simulink library "inp"  (R2021b)
settings: Solver=VariableStepAuto  StartTime=0.0  StopTime=10.0  RelTol=1e-3
undefined symbols (not defined in the file): C_TASK_5MS_S, FALSE, KINP_AcoreReadyToSlp_flg_ovrdflg, KINP_AcoreReadyToSlp_flg_ovrdval, KINP_AllowMovThd_OTA_enum_ovrdflg, KINP_AllowMovThd_OTA_enum_ovrdval, KINP_APSAngleTarget_Deg_ovrdflg, KINP_APSAngleTarget_Deg_ovrdval, KINP_APSDecReq_mps2_ovrdflg, KINP_APSDecReq_mps2_ovrdval, KINP_APSDecReqA_flg_ovrdflg, KINP_APSDecReqA_flg_ovrdval, KINP_APSDFLL_cm_ovrdflg, KINP_APSDFLL_cm_ovrdval, KINP_APSDFLR_cm_ovrdflg, KINP_APSDFLR_cm_ovrdval, KINP_APSDRLL_cm_ovrdflg, KINP_APSDRLL_cm_ovrdval, KINP_APSDRLR_cm_ovrdflg, KINP_APSDRLR_cm_ovrdval, KINP_APSExitCondition_enum_ovrdflg, KINP_APSExitCondition_enum_ovrdval, KINP_APSHWVer_enum_ovrdflg, KINP_APSHWVer_enum_ovrdval, KINP_APSProgressPCT_pct_ovrdflg, KINP_APSProgressPCT_pct_ovrdval, KINP_APSPwrReq_enum_ovrdflg, KINP_APSPwrReq_enum_ovrdval, KINP_APSReq_enum_ovrdflg, KINP_APSReq_enum_ovrdval, KINP_APSRQDisplay_enum_ovrdflg, KINP_APSRQDisplay_enum_ovrdval, KINP_APSRqEPASCtrl_flg_ovrdflg, KINP_APSRqEPASCtrl_flg_ovrdval, KINP_APSShiftPosnReq_enum_ovrdval, KINP_APSShiftPosnReq_enum_ovrflg, KINP_APSSpeedCMD_kph_ovrdval, KINP_APSSpeedCMD_kph_ovrflg, KINP_APSStaSystem_enum_ovrdflg, KINP_APSStaSystem_enum_ovrdval, KINP_APSSWVer_enum_ovrdflg, KINP_APSSWVer_enum_ovrdval, KINP_APSVMCReqA_flg_ovrdval, KINP_APSVMCReqA_flg_ovrflg, KINP_APSVRqEPASCtrl_flg_ovrdflg, KINP_APSVRqEPASCtrl_flg_ovrdval, KINP_AuxBattVolmV_mV_ovrdflg, KINP_AuxBattVolmV_mV_ovrdval, KINP_BTConnectSta_enum_ovrdflg, KINP_BTConnectSta_enum_ovrdval, KINP_CAASSta_enum_ovrdflg, KINP_CAASSta_enum_ovrdval, KINP_CAASVMCReqA_flg_ovrdval, KINP_CAASVMCReqA_flg_ovrflg, KINP_CAN1BusOff_flg_ovrdflg, KINP_CAN1BusOff_flg_ovrdval, KINP_CAN2BusOff_flg_ovrdflg, KINP_CAN2BusOff_flg_ovrdval, KINP_CAN3BusOff_flg_ovrdflg, KINP_CAN3BusOff_flg_ovrdval ... (+158)
libraries: FVT_lib x184, hcu_lib x1
(part 4 of 8)

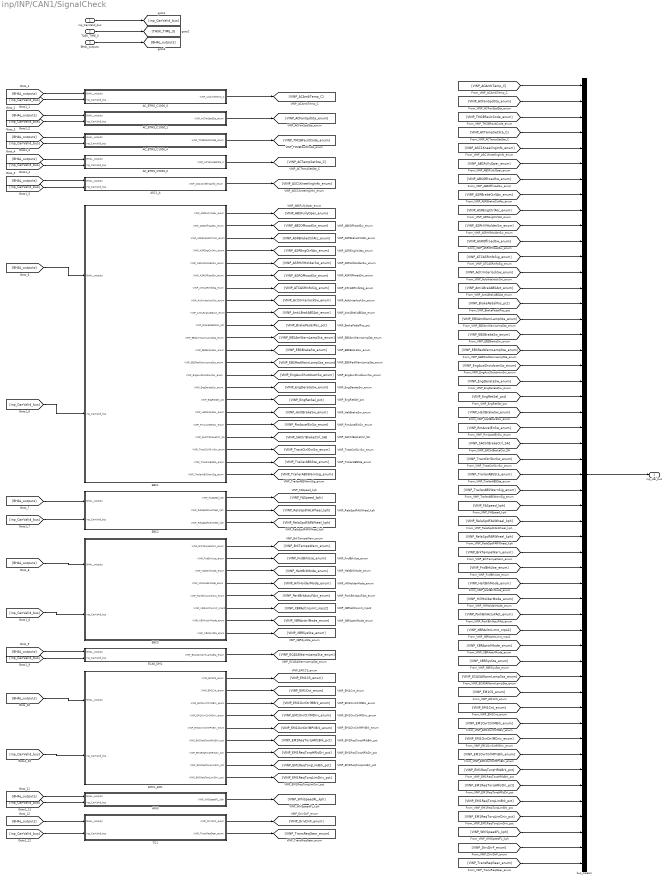
== system inp/INP/CAN1/SignalCheck ==
  inp_CanValid_bus : Inport
  TASK_TIME_S : Inport  Port=2
  BHAL_outputs : Inport  Port=3
  AC_BTMS_C1000_0 : Subsystem
  AC_BTMS_C1000_1 : Subsystem
  AC_BTMS_C1000_4 : Subsystem
  AC_BTMS_C5000_0 : Subsystem
  ASC1_A : Subsystem
  EBC1 : Subsystem
  EBC2 : Subsystem
  EBC5 : Subsystem
  ECAS_DM1 : Subsystem
  EMC1_EM1 : Subsystem
  HRW : Subsystem
  TC1 : Subsystem
  bus_creator : BusCreator  Inputs=51
  inp_Hal_bus : Outport
  wires:
  inp_CanValid_bus/1 -> [inp_CanValid_bus]
  TASK_TIME_S/1 -> [TASK_TIME_S]
  BHAL_outputs/1 -> [BHAL_outputs]
  [BHAL_outputs] -> AC_BTMS_C1000_0/1(BHAL_outputs)
  [inp_CanValid_bus] -> AC_BTMS_C1000_0/2(inp_CanValid_bus)
  AC_BTMS_C1000_0/1(VINP_ACAmbTemp_C) -> [VINP_ACAmbTemp_C]
  [BHAL_outputs] -> AC_BTMS_C1000_1/1(BHAL_outputs)
  [inp_CanValid_bus] -> AC_BTMS_C1000_1/2(inp_CanValid_bus)
  AC_BTMS_C1000_1/1(VINP_ACFanSpdSta_enum) -> [VINP_ACFanSpdSta_enum]
  [BHAL_outputs] -> AC_BTMS_C1000_4/1(BHAL_outputs)
  [inp_CanValid_bus] -> AC_BTMS_C1000_4/2(inp_CanValid_bus)
  AC_BTMS_C1000_4/1(VINP_TM2BFaultCode_enum) -> [VINP_TM2BFaultCode_enum]
  [BHAL_outputs] -> AC_BTMS_C5000_0/1(BHAL_outputs)
  [inp_CanValid_bus] -> AC_BTMS_C5000_0/2(inp_CanValid_bus)
  AC_BTMS_C5000_0/1(VINP_ACTempSetSta_C) -> [VINP_ACTempSetSta_C]
  [BHAL_outputs] -> ASC1_A/1(BHAL_outputs)
  [inp_CanValid_bus] -> ASC1_A/2(inp_CanValid_bus)
  ASC1_A/1(VINP_ASC1KneelingInfo_enum) -> [VINP_ASC1KneelingInfo_enum]
  [BHAL_outputs] -> EBC1/1(BHAL_outputs)
  [inp_CanValid_bus] -> EBC1/2(inp_CanValid_bus)
  EBC1/1(VINP_ABSFullyOper_enum) -> [VINP_ABSFullyOper_enum]
  EBC1/2(VINP_ABSOffroadSw_enum) -> [VINP_ABSOffroadSw_enum]
  EBC1/3(VINP_ASRBrakeCtrlAtc_enum) -> [VINP_ASRBrakeCtrlAtc_enum]
  EBC1/4(VINP_ASREngCtrlAtc_enum) -> [VINP_ASREngCtrlAtc_enum]
  EBC1/5(VINP_ASRHillHolderSw_enum) -> [VINP_ASRHillHolderSw_enum]
  EBC1/6(VINP_ASROffroadSw_enum) -> [VINP_ASROffroadSw_enum]
  EBC1/7(VINP_ATCASRInfoSig_enum) -> [VINP_ATCASRInfoSig_enum]
  EBC1/8(VINP_AcltrInterlockSw_enum) -> [VINP_AcltrInterlockSw_enum]
  EBC1/9(VINP_AntiLBrakABSAct_enum) -> [VINP_AntiLBrakABSAct_enum]
  EBC1/10(VINP_BrakePedalPos_pct) -> [VINP_BrakePedalPos_pct]
  EBC1/11(VINP_EBSAmWarnLampSta_enum) -> [VINP_EBSAmWarnLampSta_enum]
  EBC1/12(VINP_EBSBrakeSw_enum) -> [VINP_EBSBrakeSw_enum]
  EBC1/13(VINP_EBSRedWarnLampSta_enum) -> [VINP_EBSRedWarnLampSta_enum]
  EBC1/14(VINP_EngAuxShutdownSw_enum) -> [VINP_EngAuxShutdownSw_enum]
  EBC1/15(VINP_EngDerateSw_enum) -> [VINP_EngDerateSw_enum]
  EBC1/16(VINP_EngRetSel_pct) -> [VINP_EngRetSel_pct]
  EBC1/17(VINP_HaltBrakeSw_enum) -> [VINP_HaltBrakeSw_enum]
  EBC1/18(VINP_RmAccelEnSw_enum) -> [VINP_RmAccelEnSw_enum]
  EBC1/19(VINP_SACtrlBrakeCtrl_SA) -> [VINP_SACtrlBrakeCtrl_SA]
  EBC1/20(VINP_TractCtrlOvrSw_enum) -> [VINP_TractCtrlOvrSw_enum]
  EBC1/21(VINP_TrailerABSSta_enum) -> [VINP_TrailerABSSta_enum]
  EBC1/22(VINP_TrailerABSWarnSig_enum) -> [VINP_TrailerABSWarnSig_enum]
  [BHAL_outputs] -> EBC2/1(BHAL_outputs)
  [inp_CanValid_bus] -> EBC2/2(inp_CanValid_bus)
  EBC2/1(VINP_FASpeed_kph) -> [VINP_FASpeed_kph]
  EBC2/2(VINP_RelaSpdFALWheel_kph) -> [VINP_RelaSpdFALWheel_kph]
  EBC2/3(VINP_RelaSpdFARWheel_kph) -> [VINP_RelaSpdFARWheel_kph]
  [BHAL_outputs] -> EBC5/1(BHAL_outputs)
  [inp_CanValid_bus] -> EBC5/2(inp_CanValid_bus)
  EBC5/1(VINP_BrkTempeWarn_enum) -> [VINP_BrkTempeWarn_enum]
  EBC5/2(VINP_FndBrkUse_enum) -> [VINP_FndBrkUse_enum]
  EBC5/3(VINP_HaltBrkMode_enum) -> [VINP_HaltBrkMode_enum]
  EBC5/4(VINP_HillHolderMode_enum) -> [VINP_HillHolderMode_enum]
  EBC5/5(VINP_ParkBrkActuFAct_enum) -> [VINP_ParkBrkActuFAct_enum]
  EBC5/6(VINP_XBRAcltnLimit_mps2) -> [VINP_XBRAcltnLimit_mps2]
  EBC5/7(VINP_XBRActtrlMode_enum) -> [VINP_XBRActtrlMode_enum]
  EBC5/8(VINP_XBRSysSta_enum) -> [VINP_XBRSysSta_enum]
  [BHAL_outputs] -> ECAS_DM1/1(BHAL_outputs)
  [inp_CanValid_bus] -> ECAS_DM1/2(inp_CanValid_bus)
  ECAS_DM1/1(VINP_ECASAWarmLampSta_enum) -> [VINP_ECASAWarmLampSta_enum]
  [BHAL_outputs] -> EMC1_EM1/1(BHAL_outputs)
  [inp_CanValid_bus] -> EMC1_EM1/2(inp_CanValid_bus)
  EMC1_EM1/1(VINP_EM1CS_enum) -> [VINP_EM1CS_enum]
  EMC1_EM1/2(VINP_EM1Cnt_enum) -> [VINP_EM1Cnt_enum]
  EMC1_EM1/3(VINP_EM1OvrCtrlMBrk_enum) -> [VINP_EM1OvrCtrlMBrk_enum]
  EMC1_EM1/4(VINP_EM1OvrCtrlMDriv_enum) -> [VINP_EM1OvrCtrlMDriv_enum]
  EMC1_EM1/5(VINP_EM1OvrCtrlMPriBrk_enum) -> [VINP_EM1OvrCtrlMPriBrk_enum]
  EMC1_EM1/6(VINP_EM1ReqTorqHRlsBrk_pct) -> [VINP_EM1ReqTorqHRlsBrk_pct]
  EMC1_EM1/7(VINP_EM1ReqTorqHRlsDri_pct) -> [VINP_EM1ReqTorqHRlsDri_pct]
  EMC1_EM1/8(VINP_EM1ReqTorqLimBrk_pct) -> [VINP_EM1ReqTorqLimBrk_pct]
  EMC1_EM1/9(VINP_EM1ReqTorqLimDriv_pct) -> [VINP_EM1ReqTorqLimDriv_pct]
  [BHAL_outputs] -> HRW/1(BHAL_outputs)
  [inp_CanValid_bus] -> HRW/2(inp_CanValid_bus)
  HRW/1(VINP_WhlSpeedFL_kph) -> [VINP_WhlSpeedFL_kph]
  [BHAL_outputs] -> TC1/1(BHAL_outputs)
  [inp_CanValid_bus] -> TC1/2(inp_CanValid_bus)
  TC1/1(VINP_DrivDirF_enum) -> [VINP_DrivDirF_enum]
  TC1/2(VINP_TransReqGear_enum) -> [VINP_TransReqGear_enum]
  bus_creator/1 -> inp_Hal_bus/1
  [VINP_ACAmbTemp_C] -> bus_creator/1
  [VINP_ACFanSpdSta_enum] -> bus_creator/2
  [VINP_TM2BFaultCode_enum] -> bus_creator/3
  [VINP_ACTempSetSta_C] -> bus_creator/4
  [VINP_ASC1KneelingInfo_enum] -> bus_creator/5
  [VINP_ABSFullyOper_enum] -> bus_creator/6
  [VINP_ABSOffroadSw_enum] -> bus_creator/7
  [VINP_ASRBrakeCtrlAtc_enum] -> bus_creator/8
  [VINP_ASREngCtrlAtc_enum] -> bus_creator/9
  [VINP_ASRHillHolderSw_enum] -> bus_creator/10
  [VINP_ASROffroadSw_enum] -> bus_creator/11
  [VINP_ATCASRInfoSig_enum] -> bus_creator/12
  [VINP_AcltrInterlockSw_enum] -> bus_creator/13
  [VINP_AntiLBrakABSAct_enum] -> bus_creator/14
  [VINP_BrakePedalPos_pct] -> bus_creator/15
  [VINP_EBSAmWarnLampSta_enum] -> bus_creator/16
  [VINP_EBSBrakeSw_enum] -> bus_creator/17
  [VINP_EBSRedWarnLampSta_enum] -> bus_creator/18
  [VINP_EngAuxShutdownSw_enum] -> bus_creator/19
  [VINP_EngDerateSw_enum] -> bus_creator/20
  [VINP_EngRetSel_pct] -> bus_creator/21
  [VINP_HaltBrakeSw_enum] -> bus_creator/22
  [VINP_RmAccelEnSw_enum] -> bus_creator/23
  [VINP_SACtrlBrakeCtrl_SA] -> bus_creator/24
  [VINP_TractCtrlOvrSw_enum] -> bus_creator/25
  [VINP_TrailerABSSta_enum] -> bus_creator/26
  [VINP_TrailerABSWarnSig_enum] -> bus_creator/27
  [VINP_FASpeed_kph] -> bus_creator/28
  [VINP_RelaSpdFALWheel_kph] -> bus_creator/29
  [VINP_RelaSpdFARWheel_kph] -> bus_creator/30
  [VINP_BrkTempeWarn_enum] -> bus_creator/31
  [VINP_FndBrkUse_enum] -> bus_creator/32
  [VINP_HaltBrkMode_enum] -> bus_creator/33
  [VINP_HillHolderMode_enum] -> bus_creator/34
  [VINP_ParkBrkActuFAct_enum] -> bus_creator/35
  [VINP_XBRAcltnLimit_mps2] -> bus_creator/36
  [VINP_XBRActtrlMode_enum] -> bus_creator/37
  [VINP_XBRSysSta_enum] -> bus_creator/38
  [VINP_ECASAWarmLampSta_enum] -> bus_creator/39
  [VINP_EM1CS_enum] -> bus_creator/40
  [VINP_EM1Cnt_enum] -> bus_creator/41
  [VINP_EM1OvrCtrlMBrk_enum] -> bus_creator/42
  [VINP_EM1OvrCtrlMDriv_enum] -> bus_creator/43
  [VINP_EM1OvrCtrlMPriBrk_enum] -> bus_creator/44
  [VINP_EM1ReqTorqHRlsBrk_pct] -> bus_creator/45
  [VINP_EM1ReqTorqHRlsDri_pct] -> bus_creator/46
  [VINP_EM1ReqTorqLimBrk_pct] -> bus_creator/47
  [VINP_EM1ReqTorqLimDriv_pct] -> bus_creator/48
  [VINP_WhlSpeedFL_kph] -> bus_creator/49
  [VINP_DrivDirF_enum] -> bus_creator/50
  [VINP_TransReqGear_enum] -> bus_creator/51

== system inp/INP/CAN2/CommunicationCheck ==
  BHAL_outputs : Inport
  CANMsgInvalidIVIC1000 : FVT_lib/inp/CAN_Msg_Validity_Process_template  SystemSampleTime=-1  VariantActivationTime=update diagram  Latency=0  AutoFrameSizeCalculation=off
      link override ovrdflg: Value=KINP_CANMsgInvalidIVIC1000_flg_ovrdflg
      link override ovrdval: Value=KINP_CANMsgInvalidIVIC1000_flg_ovrdval
  bus_creator : BusCreator  Inputs=1
  bus_selector : BusSelector  OutputSignals=VHAL_CANMsgInvalidIVIC1000_flg
  not1 : Logic  Operator=NOT  AllPortsSameDT=off  OutDataTypeStr=boolean
  inp_CanValid_bus : Outport
  wires:
  BHAL_outputs/1 -> [BHAL_outputs]
  bus_selector/1 -> CANMsgInvalidIVIC1000/1  "<VHAL_CANMsgInvalidIVIC1000_flg>"
  CANMsgInvalidIVIC1000/1 -> not1/1
  not1/1 -> bus_creator/1  "VINP_CANMsgValidIVIC1000_flg"
  [BHAL_outputs] -> bus_selector/1
  bus_creator/1 -> inp_CanValid_bus/1

== system inp/INP/CAN2/CreateBus ==
  inp_CanValid_bus : Inport
  inp_Hal_bus : Inport  Port=2
  UnitConverter_1 : DataTypeConversion  OutDataTypeStr=boolean
  UnitConverter_2 : DataTypeConversion  OutDataTypeStr=uint8
  bus_creator : BusCreator  Inputs=2  OutDataTypeStr=Bus: BINP_CAN2_outputs  NonVirtualBus=on
  bus_selector : BusSelector  OutputSignals=VINP_CANMsgValidIVIC1000_flg
  bus_selector_1 : BusSelector  OutputSignals=VINP_IVIACFanSpdReqCmd_enum
  BINP_outputs : Outport
  wires:
  inp_CanValid_bus/1 -> [inp_CanValid_bus]
  inp_Hal_bus/1 -> [inp_Hal_bus]
  bus_selector/1 -> UnitConverter_1/1  "<VINP_CANMsgValidIVIC1000_flg>"
  UnitConverter_1/1 -> bus_creator/1  "VINP_CANMsgValidIVIC1000_flg"
  bus_selector_1/1 -> UnitConverter_2/1  "<VINP_IVIACFanSpdReqCmd_enum>"
  UnitConverter_2/1 -> bus_creator/2  "VINP_IVIACFanSpdReqCmd_enum"
  [inp_CanValid_bus] -> bus_selector/1
  [inp_Hal_bus] -> bus_selector_1/1
  bus_creator/1 -> BINP_outputs/1

== system inp/INP/CAN2/SignalCheck ==
  inp_CanValid_bus : Inport
  TASK_TIME_S : Inport  Port=2
  BHAL_outputs : Inport  Port=3
  IVI_C100_0 : Subsystem
  bus_creator : BusCreator  Inputs=1
  inp_Hal_bus : Outport
  wires:
  inp_CanValid_bus/1 -> [inp_CanValid_bus]
  TASK_TIME_S/1 -> [TASK_TIME_S]
  BHAL_outputs/1 -> [BHAL_outputs]
  [BHAL_outputs] -> IVI_C100_0/1(BHAL_outputs)
  [inp_CanValid_bus] -> IVI_C100_0/2(inp_CanValid_bus)
  IVI_C100_0/1(VINP_IVIACFanSpdReqCmd_enum) -> [VINP_IVIACFanSpdReqCmd_enum]
  bus_creator/1 -> inp_Hal_bus/1
  [VINP_IVIACFanSpdReqCmd_enum] -> bus_creator/1

== system inp/INP/CAN3/CommunicationCheck ==
  BHAL_outputs : Inport
  CANMsgInvalidB2TMInfo : FVT_lib/inp/CAN_Msg_Validity_Process_template  SystemSampleTime=-1  VariantActivationTime=update diagram  Latency=0  AutoFrameSizeCalculation=off
      link override ovrdflg: Value=KINP_CANMsgInvalidB2TMInfo_flg_ovrdflg
      link override ovrdval: Value=KINP_CANMsgInvalidB2TMInfo_flg_ovrdval
  CANMsgInvalidB2VBattInfo1 : FVT_lib/inp/CAN_Msg_Validity_Process_template  SystemSampleTime=-1  VariantActivationTime=update diagram  Latency=0  AutoFrameSizeCalculation=off
      link override ovrdflg: Value=KINP_CANMsgInvalidB2VBattInfo1_flg_ovrdflg
      link override ovrdval: Value=KINP_CANMsgInvalidB2VBattInfo1_flg_ovrdval
  CANMsgInvalidB2VCurrentLimit : FVT_lib/inp/CAN_Msg_Validity_Process_template  SystemSampleTime=-1  VariantActivationTime=update diagram  Latency=0  AutoFrameSizeCalculation=off
      link override ovrdflg: Value=KINP_CANMsgInvalidB2VCurrentLimit_flg_ovrdflg
      link override ovrdval: Value=KINP_CANMsgInvalidB2VCurrentLimit_flg_ovrdval
  CANMsgInvalidB2VFult132960 : FVT_lib/inp/CAN_Msg_Validity_Process_template  SystemSampleTime=-1  VariantActivationTime=update diagram  Latency=0  AutoFrameSizeCalculation=off
      link override ovrdflg: Value=KINP_CANMsgInvalidB2VFult132960_flg_ovrdflg
      link override ovrdval: Value=KINP_CANMsgInvalidB2VFult132960_flg_ovrdval
  CANMsgInvalidB2VST1 : FVT_lib/inp/CAN_Msg_Validity_Process_template  SystemSampleTime=-1  VariantActivationTime=update diagram  Latency=0  AutoFrameSizeCalculation=off
      link override ovrdflg: Value=KINP_CANMsgInvalidB2VST1_flg_ovrdflg
      link override ovrdval: Value=KINP_CANMsgInvalidB2VST1_flg_ovrdval
  CANMsgInvalidB2VST2 : FVT_lib/inp/CAN_Msg_Validity_Process_template  SystemSampleTime=-1  VariantActivationTime=update diagram  Latency=0  AutoFrameSizeCalculation=off
      link override ovrdflg: Value=KINP_CANMsgInvalidB2VST2_flg_ovrdflg
      link override ovrdval: Value=KINP_CANMsgInvalidB2VST2_flg_ovrdval
  CANMsgInvalidB2VST4 : FVT_lib/inp/CAN_Msg_Validity_Process_template  SystemSampleTime=-1  VariantActivationTime=update diagram  Latency=0  AutoFrameSizeCalculation=off
      link override ovrdflg: Value=KINP_CANMsgInvalidB2VST4_flg_ovrdflg
      link override ovrdval: Value=KINP_CANMsgInvalidB2VST4_flg_ovrdval
  CANMsgInvalidB2VST5 : FVT_lib/inp/CAN_Msg_Validity_Process_template  SystemSampleTime=-1  VariantActivationTime=update diagram  Latency=0  AutoFrameSizeCalculation=off
      link override ovrdflg: Value=KINP_CANMsgInvalidB2VST5_flg_ovrdflg
      link override ovrdval: Value=KINP_CANMsgInvalidB2VST5_flg_ovrdval
  CANMsgInvalidEWP1 : FVT_lib/inp/CAN_Msg_Validity_Process_template  SystemSampleTime=-1  VariantActivationTime=update diagram  Latency=0  AutoFrameSizeCalculation=off
      link override ovrdflg: Value=KINP_CANMsgInvalidEWP1_flg_ovrdflg
      link override ovrdval: Value=KINP_CANMsgInvalidEWP1_flg_ovrdval
  CANMsgInvalidTMMCUSta1 : FVT_lib/inp/CAN_Msg_Validity_Process_template  SystemSampleTime=-1  VariantActivationTime=update diagram  Latency=0  AutoFrameSizeCalculation=off
      link override ovrdflg: Value=KINP_CANMsgInvalidTMMCUSta1_flg_ovrdflg
      link override ovrdval: Value=KINP_CANMsgInvalidTMMCUSta1_flg_ovrdval
  CANMsgInvalidTMMCUSta2 : FVT_lib/inp/CAN_Msg_Validity_Process_template  SystemSampleTime=-1  VariantActivationTime=update diagram  Latency=0  AutoFrameSizeCalculation=off
      link override ovrdflg: Value=KINP_CANMsgInvalidTMMCUSta2_flg_ovrdflg
      link override ovrdval: Value=KINP_CANMsgInvalidTMMCUSta2_flg_ovrdval
  CANMsgInvalidTMMCUSta3 : FVT_lib/inp/CAN_Msg_Validity_Process_template  SystemSampleTime=-1  VariantActivationTime=update diagram  Latency=0  AutoFrameSizeCalculation=off
      link override ovrdflg: Value=KINP_CANMsgInvalidTMMCUSta3_flg_ovrdflg
      link override ovrdval: Value=KINP_CANMsgInvalidTMMCUSta3_flg_ovrdval
  bus_creator : BusCreator  Inputs=12
  bus_selector : BusSelector  OutputSignals=VHAL_CANMsgInvalidB2TMInfo_flg,VHAL_CANMsgInvalidB2VBattInfo1_flg,VHAL_CANMsgInvalidB2VCurrentLimit_flg,VHAL_CANMsgInvalidB2VFult132960_flg,VHAL_CANMsgInvalidB2VST1_flg,VHAL_CANMsgInvalidB2VST2_flg,VHAL_CANMsgInvalidB2VST4_flg,VHAL_CANMsgInvalidB2VST5_flg,VHAL_CANMsgInvalidEWP1_flg,VHAL_CANMsgInvalidTMMCUSta1_flg,VHAL_CANMsgInvalidTMMCUSta2_flg,VHAL_CANMsgInvalidTMMCUSta3_flg
  not{1..12} (12 alike) : Logic  Operator=NOT  AllPortsSameDT=off  OutDataTypeStr=boolean
  inp_CanValid_bus : Outport
  wires:
  BHAL_outputs/1 -> [BHAL_outputs]
  bus_selector/1 -> CANMsgInvalidB2TMInfo/1  "<VHAL_CANMsgInvalidB2TMInfo_flg>"
  CANMsgInvalidB2TMInfo/1 -> not1/1
  not1/1 -> bus_creator/1  "VINP_CANMsgValidB2TMInfo_flg"
  bus_selector/2 -> CANMsgInvalidB2VBattInfo1/1  "<VHAL_CANMsgInvalidB2VBattInfo1_flg>"
  CANMsgInvalidB2VBattInfo1/1 -> not2/1
  not2/1 -> bus_creator/2  "VINP_CANMsgValidB2VBattInfo1_flg"
  bus_selector/3 -> CANMsgInvalidB2VCurrentLimit/1  "<VHAL_CANMsgInvalidB2VCurrentLimit_flg>"
  CANMsgInvalidB2VCurrentLimit/1 -> not3/1
  not3/1 -> bus_creator/3  "VINP_CANMsgValidB2VCurrentLimit_flg"
  bus_selector/4 -> CANMsgInvalidB2VFult132960/1  "<VHAL_CANMsgInvalidB2VFult132960_flg>"
  CANMsgInvalidB2VFult132960/1 -> not4/1
  not4/1 -> bus_creator/4  "VINP_CANMsgValidB2VFult132960_flg"
  bus_selector/5 -> CANMsgInvalidB2VST1/1  "<VHAL_CANMsgInvalidB2VST1_flg>"
  CANMsgInvalidB2VST1/1 -> not5/1
  not5/1 -> bus_creator/5  "VINP_CANMsgValidB2VST1_flg"
  bus_selector/6 -> CANMsgInvalidB2VST2/1  "<VHAL_CANMsgInvalidB2VST2_flg>"
  CANMsgInvalidB2VST2/1 -> not6/1
  not6/1 -> bus_creator/6  "VINP_CANMsgValidB2VST2_flg"
  bus_selector/7 -> CANMsgInvalidB2VST4/1  "<VHAL_CANMsgInvalidB2VST4_flg>"
  CANMsgInvalidB2VST4/1 -> not7/1
  not7/1 -> bus_creator/7  "VINP_CANMsgValidB2VST4_flg"
  bus_selector/8 -> CANMsgInvalidB2VST5/1  "<VHAL_CANMsgInvalidB2VST5_flg>"
  CANMsgInvalidB2VST5/1 -> not8/1
  not8/1 -> bus_creator/8  "VINP_CANMsgValidB2VST5_flg"
  bus_selector/9 -> CANMsgInvalidEWP1/1  "<VHAL_CANMsgInvalidEWP1_flg>"
  CANMsgInvalidEWP1/1 -> not9/1
  not9/1 -> bus_creator/9  "VINP_CANMsgValidEWP1_flg"
  bus_selector/10 -> CANMsgInvalidTMMCUSta1/1  "<VHAL_CANMsgInvalidTMMCUSta1_flg>"
  CANMsgInvalidTMMCUSta1/1 -> not10/1
  not10/1 -> bus_creator/10  "VINP_CANMsgValidTMMCUSta1_flg"
  bus_selector/11 -> CANMsgInvalidTMMCUSta2/1  "<VHAL_CANMsgInvalidTMMCUSta2_flg>"
  CANMsgInvalidTMMCUSta2/1 -> not11/1
  not11/1 -> bus_creator/11  "VINP_CANMsgValidTMMCUSta2_flg"
  bus_selector/12 -> CANMsgInvalidTMMCUSta3/1  "<VHAL_CANMsgInvalidTMMCUSta3_flg>"
  CANMsgInvalidTMMCUSta3/1 -> not12/1
  not12/1 -> bus_creator/12  "VINP_CANMsgValidTMMCUSta3_flg"
  [BHAL_outputs] -> bus_selector/1
  bus_creator/1 -> inp_CanValid_bus/1

== system inp/INP/CAN3/CreateBus ==
  inp_CanValid_bus : Inport
  inp_Hal_bus : Inport  Port=2
  UnitConverter_{1..12,17..18,37,39} (16 alike) : DataTypeConversion  OutDataTypeStr=boolean
  UnitConverter_{13..14,19..29,32,34,36,38,42,49} (19 alike) : DataTypeConversion  OutDataTypeStr=uint8
  UnitConverter_{15..16,30..31,33,35,40..41,43..48} (14 alike) : DataTypeConversion  OutDataTypeStr=single
  bus_creator : BusCreator  Inputs=49  OutDataTypeStr=Bus: BINP_CAN3_outputs  NonVirtualBus=on
  bus_selector : BusSelector  OutputSignals=VINP_CANMsgValidB2TMInfo_flg,VINP_CANMsgValidB2VBattInfo1_flg,VINP_CANMsgValidB2VCurrentLimit_flg,VINP_CANMsgValidB2VFult132960_flg,VINP_CANMsgValidB2VST1_flg,VINP_CANMsgValidB2VST2_flg,VINP_CANMsgValidB2VST4_flg,VINP_CANMsgValidB2VST5_flg,VINP_CANMsgValidEWP1_flg,VINP_CANMsgValidTMMCUSta1_flg,VINP_CANMsgValidTMMCUSta2_flg,VINP_CANMsgValidTMMCUSta3_flg
  bus_selector_1 : BusSelector  OutputSignals=VINP_B2THVRlySta_enum,VINP_B2VBI1BattType_enum,VINP_B2VAPlsDischgCurr_A,VINP_B2VAvaPlsChgCurr_A,VINP_B2VHVILFault_flg,VINP_B2VACChgConnSta_flg,VINP_B2VACChgNegRlySta_enum,VINP_B2VACChgPosRlySta_enum,VINP_B2VBMUHVSta_enum,VINP_B2VChgMode_enum,VINP_B2VChgSta_enum,VINP_B2VDCChgConnSta_enum,VINP_B2VDCChgN1RlySta_enum,VINP_B2VDCChgP1RlySta_enum,VINP_B2VMainNegRlySta_enum,VINP_B2VFaultCode_enum,VINP_B2VFaultLv_enum,VINP_B2VPackCurr_A,VINP_B2VPackInsideVol_V,VINP_B2VRqHVPwrOff_enum,VINP_B2VSOC_pct,VINP_B2VMinTempPos_enum,VINP_B2VCellMinVol_V,VINP_EWPPEFault_enum,VINP_AtvDisChgEnFbk_flg,VINP_MCUCtrlMdSta_enum,VINP_MCUIGBTEnFbk_flg,VINP_MotorSpd_rpm,VINP_MotorTrq_Nm,VINP_MCUFailGrade_enum,VINP_MCUTemp_C,VINP_MCUTrqLimHi_Nm,VINP_MCUTrqLimLo_Nm,VINP_MotorTemp_C,VINP_MCUDCCur_A,VINP_MCUDCVol_V,VINP_MCUFailCode_enum
  BINP_outputs : Outport
  wires:
  inp_CanValid_bus/1 -> [inp_CanValid_bus]
  inp_Hal_bus/1 -> [inp_Hal_bus]
  bus_selector/1 -> UnitConverter_1/1  "<VINP_CANMsgValidB2TMInfo_flg>"
  UnitConverter_1/1 -> bus_creator/1  "VINP_CANMsgValidB2TMInfo_flg"
  bus_selector/2 -> UnitConverter_2/1  "<VINP_CANMsgValidB2VBattInfo1_flg>"
  UnitConverter_2/1 -> bus_creator/2  "VINP_CANMsgValidB2VBattInfo1_flg"
  bus_selector/3 -> UnitConverter_3/1  "<VINP_CANMsgValidB2VCurrentLimit_flg>"
  UnitConverter_3/1 -> bus_creator/3  "VINP_CANMsgValidB2VCurrentLimit_flg"
  bus_selector/4 -> UnitConverter_4/1  "<VINP_CANMsgValidB2VFult132960_flg>"
  UnitConverter_4/1 -> bus_creator/4  "VINP_CANMsgValidB2VFult132960_flg"
  bus_selector/5 -> UnitConverter_5/1  "<VINP_CANMsgValidB2VST1_flg>"
  UnitConverter_5/1 -> bus_creator/5  "VINP_CANMsgValidB2VST1_flg"
  bus_selector/6 -> UnitConverter_6/1  "<VINP_CANMsgValidB2VST2_flg>"
  UnitConverter_6/1 -> bus_creator/6  "VINP_CANMsgValidB2VST2_flg"
  bus_selector/7 -> UnitConverter_7/1  "<VINP_CANMsgValidB2VST4_flg>"
  UnitConverter_7/1 -> bus_creator/7  "VINP_CANMsgValidB2VST4_flg"
  bus_selector/8 -> UnitConverter_8/1  "<VINP_CANMsgValidB2VST5_flg>"
  UnitConverter_8/1 -> bus_creator/8  "VINP_CANMsgValidB2VST5_flg"
  bus_selector/9 -> UnitConverter_9/1  "<VINP_CANMsgValidEWP1_flg>"
  UnitConverter_9/1 -> bus_creator/9  "VINP_CANMsgValidEWP1_flg"
  bus_selector/10 -> UnitConverter_10/1  "<VINP_CANMsgValidTMMCUSta1_flg>"
  UnitConverter_10/1 -> bus_creator/10  "VINP_CANMsgValidTMMCUSta1_flg"
  bus_selector/11 -> UnitConverter_11/1  "<VINP_CANMsgValidTMMCUSta2_flg>"
  UnitConverter_11/1 -> bus_creator/11  "VINP_CANMsgValidTMMCUSta2_flg"
  bus_selector/12 -> UnitConverter_12/1  "<VINP_CANMsgValidTMMCUSta3_flg>"
  UnitConverter_12/1 -> bus_creator/12  "VINP_CANMsgValidTMMCUSta3_flg"
  bus_selector_1/1 -> UnitConverter_13/1  "<VINP_B2THVRlySta_enum>"
  UnitConverter_13/1 -> bus_creator/13  "VINP_B2THVRlySta_enum"
  bus_selector_1/2 -> UnitConverter_14/1  "<VINP_B2VBI1BattType_enum>"
  UnitConverter_14/1 -> bus_creator/14  "VINP_B2VBI1BattType_enum"
  bus_selector_1/3 -> UnitConverter_15/1  "<VINP_B2VAPlsDischgCurr_A>"
  UnitConverter_15/1 -> bus_creator/15  "VINP_B2VAPlsDischgCurr_A"
  bus_selector_1/4 -> UnitConverter_16/1  "<VINP_B2VAvaPlsChgCurr_A>"
  UnitConverter_16/1 -> bus_creator/16  "VINP_B2VAvaPlsChgCurr_A"
  bus_selector_1/5 -> UnitConverter_17/1  "<VINP_B2VHVILFault_flg>"
  UnitConverter_17/1 -> bus_creator/17  "VINP_B2VHVILFault_flg"
  bus_selector_1/6 -> UnitConverter_18/1  "<VINP_B2VACChgConnSta_flg>"
  UnitConverter_18/1 -> bus_creator/18  "VINP_B2VACChgConnSta_flg"
  bus_selector_1/7 -> UnitConverter_19/1  "<VINP_B2VACChgNegRlySta_enum>"
  UnitConverter_19/1 -> bus_creator/19  "VINP_B2VACChgNegRlySta_enum"
  bus_selector_1/8 -> UnitConverter_20/1  "<VINP_B2VACChgPosRlySta_enum>"
  UnitConverter_20/1 -> bus_creator/20  "VINP_B2VACChgPosRlySta_enum"
  bus_selector_1/9 -> UnitConverter_21/1  "<VINP_B2VBMUHVSta_enum>"
  UnitConverter_21/1 -> bus_creator/21  "VINP_B2VBMUHVSta_enum"
  bus_selector_1/10 -> UnitConverter_22/1  "<VINP_B2VChgMode_enum>"
  UnitConverter_22/1 -> bus_creator/22  "VINP_B2VChgMode_enum"
  bus_selector_1/11 -> UnitConverter_23/1  "<VINP_B2VChgSta_enum>"
  UnitConverter_23/1 -> bus_creator/23  "VINP_B2VChgSta_enum"
  bus_selector_1/12 -> UnitConverter_24/1  "<VINP_B2VDCChgConnSta_enum>"
  UnitConverter_24/1 -> bus_creator/24  "VINP_B2VDCChgConnSta_enum"
  bus_selector_1/13 -> UnitConverter_25/1  "<VINP_B2VDCChgN1RlySta_enum>"
  UnitConverter_25/1 -> bus_creator/25  "VINP_B2VDCChgN1RlySta_enum"
  bus_selector_1/14 -> UnitConverter_26/1  "<VINP_B2VDCChgP1RlySta_enum>"
  UnitConverter_26/1 -> bus_creator/26  "VINP_B2VDCChgP1RlySta_enum"
  bus_selector_1/15 -> UnitConverter_27/1  "<VINP_B2VMainNegRlySta_enum>"
  UnitConverter_27/1 -> bus_creator/27  "VINP_B2VMainNegRlySta_enum"
  bus_selector_1/16 -> UnitConverter_28/1  "<VINP_B2VFaultCode_enum>"
  UnitConverter_28/1 -> bus_creator/28  "VINP_B2VFaultCode_enum"
  bus_selector_1/17 -> UnitConverter_29/1  "<VINP_B2VFaultLv_enum>"
  UnitConverter_29/1 -> bus_creator/29  "VINP_B2VFaultLv_enum"
  bus_selector_1/18 -> UnitConverter_30/1  "<VINP_B2VPackCurr_A>"
  UnitConverter_30/1 -> bus_creator/30  "VINP_B2VPackCurr_A"
  bus_selector_1/19 -> UnitConverter_31/1  "<VINP_B2VPackInsideVol_V>"
  UnitConverter_31/1 -> bus_creator/31  "VINP_B2VPackInsideVol_V"
  bus_selector_1/20 -> UnitConverter_32/1  "<VINP_B2VRqHVPwrOff_enum>"
  UnitConverter_32/1 -> bus_creator/32  "VINP_B2VRqHVPwrOff_enum"
  bus_selector_1/21 -> UnitConverter_33/1  "<VINP_B2VSOC_pct>"
  UnitConverter_33/1 -> bus_creator/33  "VINP_B2VSOC_pct"
  bus_selector_1/22 -> UnitConverter_34/1  "<VINP_B2VMinTempPos_enum>"
  UnitConverter_34/1 -> bus_creator/34  "VINP_B2VMinTempPos_enum"
  bus_selector_1/23 -> UnitConverter_35/1  "<VINP_B2VCellMinVol_V>"
  UnitConverter_35/1 -> bus_creator/35  "VINP_B2VCellMinVol_V"
  bus_selector_1/24 -> UnitConverter_36/1  "<VINP_EWPPEFault_enum>"
  UnitConverter_36/1 -> bus_creator/36  "VINP_EWPPEFault_enum"
  bus_selector_1/25 -> UnitConverter_37/1  "<VINP_AtvDisChgEnFbk_flg>"
  UnitConverter_37/1 -> bus_creator/37  "VINP_AtvDisChgEnFbk_flg"
  bus_selector_1/26 -> UnitConverter_38/1  "<VINP_MCUCtrlMdSta_enum>"
  UnitConverter_38/1 -> bus_creator/38  "VINP_MCUCtrlMdSta_enum"
  bus_selector_1/27 -> UnitConverter_39/1  "<VINP_MCUIGBTEnFbk_flg>"
  UnitConverter_39/1 -> bus_creator/39  "VINP_MCUIGBTEnFbk_flg"
  bus_selector_1/28 -> UnitConverter_40/1  "<VINP_MotorSpd_rpm>"
  UnitConverter_40/1 -> bus_creator/40  "VINP_MotorSpd_rpm"
  bus_selector_1/29 -> UnitConverter_41/1  "<VINP_MotorTrq_Nm>"
  UnitConverter_41/1 -> bus_creator/41  "VINP_MotorTrq_Nm"
  bus_selector_1/30 -> UnitConverter_42/1  "<VINP_MCUFailGrade_enum>"
  UnitConverter_42/1 -> bus_creator/42  "VINP_MCUFailGrade_enum"
  bus_selector_1/31 -> UnitConverter_43/1  "<VINP_MCUTemp_C>"
  UnitConverter_43/1 -> bus_creator/43  "VINP_MCUTemp_C"
  bus_selector_1/32 -> UnitConverter_44/1  "<VINP_MCUTrqLimHi_Nm>"
  UnitConverter_44/1 -> bus_creator/44  "VINP_MCUTrqLimHi_Nm"
  bus_selector_1/33 -> UnitConverter_45/1  "<VINP_MCUTrqLimLo_Nm>"
  UnitConverter_45/1 -> bus_creator/45  "VINP_MCUTrqLimLo_Nm"
  bus_selector_1/34 -> UnitConverter_46/1  "<VINP_MotorTemp_C>"
  UnitConverter_46/1 -> bus_creator/46  "VINP_MotorTemp_C"
  bus_selector_1/35 -> UnitConverter_47/1  "<VINP_MCUDCCur_A>"
  UnitConverter_47/1 -> bus_creator/47  "VINP_MCUDCCur_A"
  bus_selector_1/36 -> UnitConverter_48/1  "<VINP_MCUDCVol_V>"
  UnitConverter_48/1 -> bus_creator/48  "VINP_MCUDCVol_V"
  bus_selector_1/37 -> UnitConverter_49/1  "<VINP_MCUFailCode_enum>"
  UnitConverter_49/1 -> bus_creator/49  "VINP_MCUFailCode_enum"
  [inp_CanValid_bus] -> bus_selector/1
  [inp_Hal_bus] -> bus_selector_1/1
  bus_creator/1 -> BINP_outputs/1

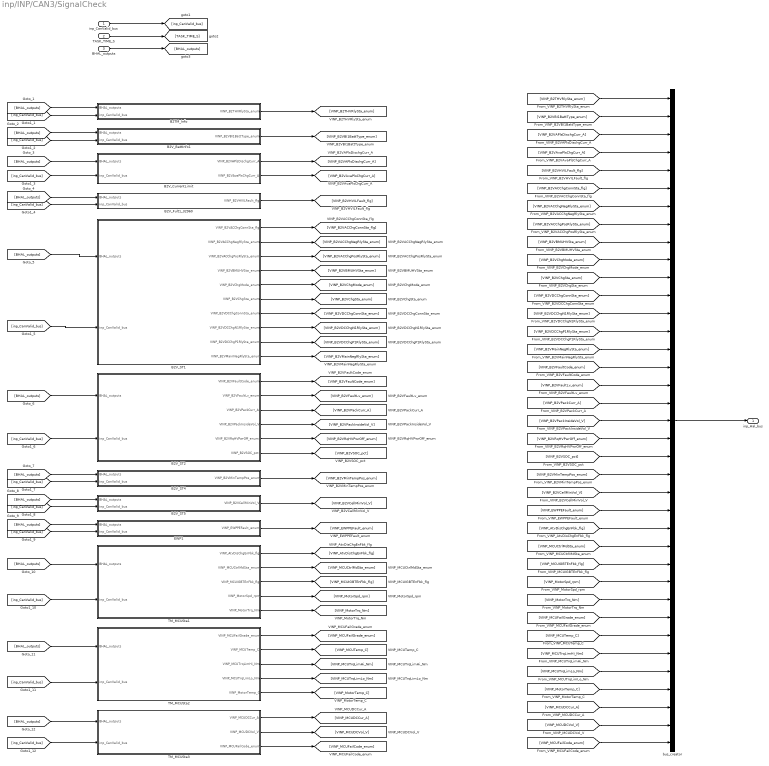
== system inp/INP/CAN3/SignalCheck ==
  inp_CanValid_bus : Inport
  TASK_TIME_S : Inport  Port=2
  BHAL_outputs : Inport  Port=3
  B2TM_Info : Subsystem
  B2V_BattInfo1 : Subsystem
  B2V_CurrentLimit : Subsystem
  B2V_Fult1_32960 : Subsystem
  B2V_ST1 : Subsystem
  B2V_ST2 : Subsystem
  B2V_ST4 : Subsystem
  B2V_ST5 : Subsystem
  EWP1 : Subsystem
  TM_MCUSta1 : Subsystem
  TM_MCUSta2 : Subsystem
  TM_MCUSta3 : Subsystem
  bus_creator : BusCreator  Inputs=37
  inp_Hal_bus : Outport
  wires:
  inp_CanValid_bus/1 -> [inp_CanValid_bus]
  TASK_TIME_S/1 -> [TASK_TIME_S]
  BHAL_outputs/1 -> [BHAL_outputs]
  [BHAL_outputs] -> B2TM_Info/1(BHAL_outputs)
  [inp_CanValid_bus] -> B2TM_Info/2(inp_CanValid_bus)
  B2TM_Info/1(VINP_B2THVRlySta_enum) -> [VINP_B2THVRlySta_enum]
  [BHAL_outputs] -> B2V_BattInfo1/1(BHAL_outputs)
  [inp_CanValid_bus] -> B2V_BattInfo1/2(inp_CanValid_bus)
  B2V_BattInfo1/1(VINP_B2VBI1BattType_enum) -> [VINP_B2VBI1BattType_enum]
  [BHAL_outputs] -> B2V_CurrentLimit/1(BHAL_outputs)
  [inp_CanValid_bus] -> B2V_CurrentLimit/2(inp_CanValid_bus)
  B2V_CurrentLimit/1(VINP_B2VAPlsDischgCurr_A) -> [VINP_B2VAPlsDischgCurr_A]
  B2V_CurrentLimit/2(VINP_B2VAvaPlsChgCurr_A) -> [VINP_B2VAvaPlsChgCurr_A]
  [BHAL_outputs] -> B2V_Fult1_32960/1(BHAL_outputs)
  [inp_CanValid_bus] -> B2V_Fult1_32960/2(inp_CanValid_bus)
  B2V_Fult1_32960/1(VINP_B2VHVILFault_flg) -> [VINP_B2VHVILFault_flg]
  [BHAL_outputs] -> B2V_ST1/1(BHAL_outputs)
  [inp_CanValid_bus] -> B2V_ST1/2(inp_CanValid_bus)
  B2V_ST1/1(VINP_B2VACChgConnSta_flg) -> [VINP_B2VACChgConnSta_flg]
  B2V_ST1/2(VINP_B2VACChgNegRlySta_enum) -> [VINP_B2VACChgNegRlySta_enum]
  B2V_ST1/3(VINP_B2VACChgPosRlySta_enum) -> [VINP_B2VACChgPosRlySta_enum]
  B2V_ST1/4(VINP_B2VBMUHVSta_enum) -> [VINP_B2VBMUHVSta_enum]
  B2V_ST1/5(VINP_B2VChgMode_enum) -> [VINP_B2VChgMode_enum]
  B2V_ST1/6(VINP_B2VChgSta_enum) -> [VINP_B2VChgSta_enum]
  B2V_ST1/7(VINP_B2VDCChgConnSta_enum) -> [VINP_B2VDCChgConnSta_enum]
  B2V_ST1/8(VINP_B2VDCChgN1RlySta_enum) -> [VINP_B2VDCChgN1RlySta_enum]
  B2V_ST1/9(VINP_B2VDCChgP1RlySta_enum) -> [VINP_B2VDCChgP1RlySta_enum]
  B2V_ST1/10(VINP_B2VMainNegRlySta_enum) -> [VINP_B2VMainNegRlySta_enum]
  [BHAL_outputs] -> B2V_ST2/1(BHAL_outputs)
  [inp_CanValid_bus] -> B2V_ST2/2(inp_CanValid_bus)
  B2V_ST2/1(VINP_B2VFaultCode_enum) -> [VINP_B2VFaultCode_enum]
  B2V_ST2/2(VINP_B2VFaultLv_enum) -> [VINP_B2VFaultLv_enum]
  B2V_ST2/3(VINP_B2VPackCurr_A) -> [VINP_B2VPackCurr_A]
  B2V_ST2/4(VINP_B2VPackInsideVol_V) -> [VINP_B2VPackInsideVol_V]
  B2V_ST2/5(VINP_B2VRqHVPwrOff_enum) -> [VINP_B2VRqHVPwrOff_enum]
  B2V_ST2/6(VINP_B2VSOC_pct) -> [VINP_B2VSOC_pct]
  [BHAL_outputs] -> B2V_ST4/1(BHAL_outputs)
  [inp_CanValid_bus] -> B2V_ST4/2(inp_CanValid_bus)
  B2V_ST4/1(VINP_B2VMinTempPos_enum) -> [VINP_B2VMinTempPos_enum]
  [BHAL_outputs] -> B2V_ST5/1(BHAL_outputs)
  [inp_CanValid_bus] -> B2V_ST5/2(inp_CanValid_bus)
  B2V_ST5/1(VINP_B2VCellMinVol_V) -> [VINP_B2VCellMinVol_V]
  [BHAL_outputs] -> EWP1/1(BHAL_outputs)
  [inp_CanValid_bus] -> EWP1/2(inp_CanValid_bus)
  EWP1/1(VINP_EWPPEFault_enum) -> [VINP_EWPPEFault_enum]
  [BHAL_outputs] -> TM_MCUSta1/1(BHAL_outputs)
  [inp_CanValid_bus] -> TM_MCUSta1/2(inp_CanValid_bus)
  TM_MCUSta1/1(VINP_AtvDisChgEnFbk_flg) -> [VINP_AtvDisChgEnFbk_flg]
  TM_MCUSta1/2(VINP_MCUCtrlMdSta_enum) -> [VINP_MCUCtrlMdSta_enum]
  TM_MCUSta1/3(VINP_MCUIGBTEnFbk_flg) -> [VINP_MCUIGBTEnFbk_flg]
  TM_MCUSta1/4(VINP_MotorSpd_rpm) -> [VINP_MotorSpd_rpm]
  TM_MCUSta1/5(VINP_MotorTrq_Nm) -> [VINP_MotorTrq_Nm]
  [BHAL_outputs] -> TM_MCUSta2/1(BHAL_outputs)
  [inp_CanValid_bus] -> TM_MCUSta2/2(inp_CanValid_bus)
  TM_MCUSta2/1(VINP_MCUFailGrade_enum) -> [VINP_MCUFailGrade_enum]
  TM_MCUSta2/2(VINP_MCUTemp_C) -> [VINP_MCUTemp_C]
  TM_MCUSta2/3(VINP_MCUTrqLimHi_Nm) -> [VINP_MCUTrqLimHi_Nm]
  TM_MCUSta2/4(VINP_MCUTrqLimLo_Nm) -> [VINP_MCUTrqLimLo_Nm]
  TM_MCUSta2/5(VINP_MotorTemp_C) -> [VINP_MotorTemp_C]
  [BHAL_outputs] -> TM_MCUSta3/1(BHAL_outputs)
  [inp_CanValid_bus] -> TM_MCUSta3/2(inp_CanValid_bus)
  TM_MCUSta3/1(VINP_MCUDCCur_A) -> [VINP_MCUDCCur_A]
  TM_MCUSta3/2(VINP_MCUDCVol_V) -> [VINP_MCUDCVol_V]
  TM_MCUSta3/3(VINP_MCUFailCode_enum) -> [VINP_MCUFailCode_enum]
  bus_creator/1 -> inp_Hal_bus/1
  [VINP_B2THVRlySta_enum] -> bus_creator/1
  [VINP_B2VBI1BattType_enum] -> bus_creator/2
  [VINP_B2VAPlsDischgCurr_A] -> bus_creator/3
  [VINP_B2VAvaPlsChgCurr_A] -> bus_creator/4
  [VINP_B2VHVILFault_flg] -> bus_creator/5
  [VINP_B2VACChgConnSta_flg] -> bus_creator/6
  [VINP_B2VACChgNegRlySta_enum] -> bus_creator/7
  [VINP_B2VACChgPosRlySta_enum] -> bus_creator/8
  [VINP_B2VBMUHVSta_enum] -> bus_creator/9
  [VINP_B2VChgMode_enum] -> bus_creator/10
  [VINP_B2VChgSta_enum] -> bus_creator/11
  [VINP_B2VDCChgConnSta_enum] -> bus_creator/12
  [VINP_B2VDCChgN1RlySta_enum] -> bus_creator/13
  [VINP_B2VDCChgP1RlySta_enum] -> bus_creator/14
  [VINP_B2VMainNegRlySta_enum] -> bus_creator/15
  [VINP_B2VFaultCode_enum] -> bus_creator/16
  [VINP_B2VFaultLv_enum] -> bus_creator/17
  [VINP_B2VPackCurr_A] -> bus_creator/18
  [VINP_B2VPackInsideVol_V] -> bus_creator/19
  [VINP_B2VRqHVPwrOff_enum] -> bus_creator/20
  [VINP_B2VSOC_pct] -> bus_creator/21
  [VINP_B2VMinTempPos_enum] -> bus_creator/22
  [VINP_B2VCellMinVol_V] -> bus_creator/23
  [VINP_EWPPEFault_enum] -> bus_creator/24
  [VINP_AtvDisChgEnFbk_flg] -> bus_creator/25
  [VINP_MCUCtrlMdSta_enum] -> bus_creator/26
  [VINP_MCUIGBTEnFbk_flg] -> bus_creator/27
  [VINP_MotorSpd_rpm] -> bus_creator/28
  [VINP_MotorTrq_Nm] -> bus_creator/29
  [VINP_MCUFailGrade_enum] -> bus_creator/30
  [VINP_MCUTemp_C] -> bus_creator/31
  [VINP_MCUTrqLimHi_Nm] -> bus_creator/32
  [VINP_MCUTrqLimLo_Nm] -> bus_creator/33
  [VINP_MotorTemp_C] -> bus_creator/34
  [VINP_MCUDCCur_A] -> bus_creator/35
  [VINP_MCUDCVol_V] -> bus_creator/36
  [VINP_MCUFailCode_enum] -> bus_creator/37

== system inp/INP/CAN4/CommunicationCheck ==
  BHAL_outputs : Inport
  CANMsgInvalidZFRC1000 : FVT_lib/inp/CAN_Msg_Validity_Process_template  SystemSampleTime=-1  VariantActivationTime=update diagram  Latency=0  AutoFrameSizeCalculation=off
      link override ovrdflg: Value=KINP_CANMsgInvalidZFRC1000_flg_ovrdflg
      link override ovrdval: Value=KINP_CANMsgInvalidZFRC1000_flg_ovrdval
  CANMsgInvalidZFRCE1000 : FVT_lib/inp/CAN_Msg_Validity_Process_template  SystemSampleTime=-1  VariantActivationTime=update diagram  Latency=0  AutoFrameSizeCalculation=off
      link override ovrdflg: Value=KINP_CANMsgInvalidZFRCE1000_flg_ovrdflg
      link override ovrdval: Value=KINP_CANMsgInvalidZFRCE1000_flg_ovrdval
  CANMsgInvalidZRRCE1000 : FVT_lib/inp/CAN_Msg_Validity_Process_template  SystemSampleTime=-1  VariantActivationTime=update diagram  Latency=0  AutoFrameSizeCalculation=off
      link override ovrdflg: Value=KINP_CANMsgInvalidZRRCE1000_flg_ovrdflg
      link override ovrdval: Value=KINP_CANMsgInvalidZRRCE1000_flg_ovrdval
  CANMsgInvalidZRRCE1001 : FVT_lib/inp/CAN_Msg_Validity_Process_template  SystemSampleTime=-1  VariantActivationTime=update diagram  Latency=0  AutoFrameSizeCalculation=off
      link override ovrdflg: Value=KINP_CANMsgInvalidZRRCE1001_flg_ovrdflg
      link override ovrdval: Value=KINP_CANMsgInvalidZRRCE1001_flg_ovrdval
  CANMsgInvalidzGWCANRr1C500 : FVT_lib/inp/CAN_Msg_Validity_Process_template  SystemSampleTime=-1  VariantActivationTime=update diagram  Latency=0  AutoFrameSizeCalculation=off
      link override ovrdflg: Value=KINP_CANMsgInvalidzGWCANRr1C500_flg_ovrdflg
      link override ovrdval: Value=KINP_CANMsgInvalidzGWCANRr1C500_flg_ovrdval
  bus_creator : BusCreator  Inputs=5
  bus_selector : BusSelector  OutputSignals=VHAL_CANMsgInvalidZFRC1000_flg,VHAL_CANMsgInvalidZFRCE1000_flg,VHAL_CANMsgInvalidZRRCE1000_flg,VHAL_CANMsgInvalidZRRCE1001_flg,VHAL_CANMsgInvalidzGWCANRr1C500_flg
  not{1..5} (5 alike) : Logic  Operator=NOT  AllPortsSameDT=off  OutDataTypeStr=boolean
  inp_CanValid_bus : Outport
  wires:
  BHAL_outputs/1 -> [BHAL_outputs]
  bus_selector/1 -> CANMsgInvalidZFRC1000/1  "<VHAL_CANMsgInvalidZFRC1000_flg>"
  CANMsgInvalidZFRC1000/1 -> not1/1
  not1/1 -> bus_creator/1  "VINP_CANMsgValidZFRC1000_flg"
  bus_selector/2 -> CANMsgInvalidZFRCE1000/1  "<VHAL_CANMsgInvalidZFRCE1000_flg>"
  CANMsgInvalidZFRCE1000/1 -> not2/1
  not2/1 -> bus_creator/2  "VINP_CANMsgValidZFRCE1000_flg"
  bus_selector/3 -> CANMsgInvalidZRRCE1000/1  "<VHAL_CANMsgInvalidZRRCE1000_flg>"
  CANMsgInvalidZRRCE1000/1 -> not3/1
  not3/1 -> bus_creator/3  "VINP_CANMsgValidZRRCE1000_flg"
  bus_selector/4 -> CANMsgInvalidZRRCE1001/1  "<VHAL_CANMsgInvalidZRRCE1001_flg>"
  CANMsgInvalidZRRCE1001/1 -> not4/1
  not4/1 -> bus_creator/4  "VINP_CANMsgValidZRRCE1001_flg"
  bus_selector/5 -> CANMsgInvalidzGWCANRr1C500/1  "<VHAL_CANMsgInvalidzGWCANRr1C500_flg>"
  CANMsgInvalidzGWCANRr1C500/1 -> not5/1
  not5/1 -> bus_creator/5  "VINP_CANMsgValidzGWCANRr1C500_flg"
  [BHAL_outputs] -> bus_selector/1
  bus_creator/1 -> inp_CanValid_bus/1

== system inp/INP/CAN4/CreateBus ==
  inp_CanValid_bus : Inport
  inp_Hal_bus : Inport  Port=2
  UnitConverter_{1..5,8..11,14,16..21,25..26,28,30..31} (21 alike) : DataTypeConversion  OutDataTypeStr=boolean
  UnitConverter_{7,12..13,15,23..24,27,29,34..35,38,41..42} (13 alike) : DataTypeConversion  OutDataTypeStr=single
  UnitConverter_{6,22,32..33,36..37,39..40,43..51} (17 alike) : DataTypeConversion  OutDataTypeStr=uint8
  bus_creator : BusCreator  Inputs=51  OutDataTypeStr=Bus: BINP_CAN4_outputs  NonVirtualBus=on
  bus_selector : BusSelector  OutputSignals=VINP_CANMsgValidZFRC1000_flg,VINP_CANMsgValidZFRCE1000_flg,VINP_CANMsgValidZRRCE1000_flg,VINP_CANMsgValidZRRCE1001_flg,VINP_CANMsgValidzGWCANRr1C500_flg
  bus_selector_1 : BusSelector  OutputSignals=VINP_ParkBrakeSW_enum,VINP_AirPressureFC2_kPa,VINP_ZFRBCMAutoLightSWSta_flg,VINP_ZFRBCMBrakeSta_flg,VINP_ZFRBCMHBeamSWSta_flg,VINP_ZFRBCMHeadLpSWSta_flg,VINP_ZFRBCMLFTurnLpCSta_A,VINP_ZFRBCMLightSensorVSta_V,VINP_ZFRBCMPLampSta_flg,VINP_ZFRBCMRFTurnLpCSta_A,VINP_ZFRBCMRFogLpSWSta_flg,VINP_ZFRBCMSeatbeltSta_flg,VINP_ZFRBCMWasherSWSta_flg,VINP_ZFRBCMWiperASSta_flg,VINP_ZFRBCMWiperHSWSta_flg,VINP_ZFRBCMWiperLSWSta_flg,VINP_ZRRBCMAllDoorSta_enum,VINP_AirPressurePC3_kPa,VINP_AirPressureRC1_kPa,VINP_FDCCHASSISVCUEACPressSta_flg,VINP_ZRRBCMCallingSWSta_flg,VINP_ZRRBCMLRTurnLpCSta_A,VINP_ZRRBCMPLampSta_flg,VINP_ZRRBCMRRTurnLpCSta_A,VINP_ZRRBCMSTOPSW2Sta_flg,VINP_ZRRBCMSTOPSWSta_flg,VINP_DCDCEnSta_enum,VINP_DCDCErrLvSta_enum,VINP_DCDCOutVolSta_V,VINP_DCDCTempSta_C,VINP_EACEnSta_enum,VINP_EACErrLvSta_enum,VINP_EACInvTempSta_C,VINP_EHPSEnSta_enum,VINP_EHPSErrLvSta_enum,VINP_EHPSInvTempSta_C,VINP_EHPSMotorSpdSta_rpm,VINP_PDUACRlySta_enum,VINP_PDUDCDCEACEHPSHVLoopSta_enum,VINP_PDUDCDCEACEHPSPreRlySta_enum,VINP_PDUDCDCEACEHPSRlySta_enum,VINP_PDUHVILSta_enum,VINP_PDUMCUHVLoopSta_enum,VINP_PDUMCUPosRlySta_enum,VINP_PDUMCUPreRlySta_enum,VINP_PDUSelfChkSta_enum
  BINP_outputs : Outport
  wires:
  inp_CanValid_bus/1 -> [inp_CanValid_bus]
  inp_Hal_bus/1 -> [inp_Hal_bus]
  bus_selector/1 -> UnitConverter_1/1  "<VINP_CANMsgValidZFRC1000_flg>"
  UnitConverter_1/1 -> bus_creator/1  "VINP_CANMsgValidZFRC1000_flg"
  bus_selector/2 -> UnitConverter_2/1  "<VINP_CANMsgValidZFRCE1000_flg>"
  UnitConverter_2/1 -> bus_creator/2  "VINP_CANMsgValidZFRCE1000_flg"
  bus_selector/3 -> UnitConverter_3/1  "<VINP_CANMsgValidZRRCE1000_flg>"
  UnitConverter_3/1 -> bus_creator/3  "VINP_CANMsgValidZRRCE1000_flg"
  bus_selector/4 -> UnitConverter_4/1  "<VINP_CANMsgValidZRRCE1001_flg>"
  UnitConverter_4/1 -> bus_creator/4  "VINP_CANMsgValidZRRCE1001_flg"
  bus_selector/5 -> UnitConverter_5/1  "<VINP_CANMsgValidzGWCANRr1C500_flg>"
  UnitConverter_5/1 -> bus_creator/5  "VINP_CANMsgValidzGWCANRr1C500_flg"
  bus_selector_1/1 -> UnitConverter_6/1  "<VINP_ParkBrakeSW_enum>"
  UnitConverter_6/1 -> bus_creator/6  "VINP_ParkBrakeSW_enum"
  bus_selector_1/2 -> UnitConverter_7/1  "<VINP_AirPressureFC2_kPa>"
  UnitConverter_7/1 -> bus_creator/7  "VINP_AirPressureFC2_kPa"
  bus_selector_1/3 -> UnitConverter_8/1  "<VINP_ZFRBCMAutoLightSWSta_flg>"
  UnitConverter_8/1 -> bus_creator/8  "VINP_ZFRBCMAutoLightSWSta_flg"
  bus_selector_1/4 -> UnitConverter_9/1  "<VINP_ZFRBCMBrakeSta_flg>"
  UnitConverter_9/1 -> bus_creator/9  "VINP_ZFRBCMBrakeSta_flg"
  bus_selector_1/5 -> UnitConverter_10/1  "<VINP_ZFRBCMHBeamSWSta_flg>"
  UnitConverter_10/1 -> bus_creator/10  "VINP_ZFRBCMHBeamSWSta_flg"
  bus_selector_1/6 -> UnitConverter_11/1  "<VINP_ZFRBCMHeadLpSWSta_flg>"
  UnitConverter_11/1 -> bus_creator/11  "VINP_ZFRBCMHeadLpSWSta_flg"
  bus_selector_1/7 -> UnitConverter_12/1  "<VINP_ZFRBCMLFTurnLpCSta_A>"
  UnitConverter_12/1 -> bus_creator/12  "VINP_ZFRBCMLFTurnLpCSta_A"
  bus_selector_1/8 -> UnitConverter_13/1  "<VINP_ZFRBCMLightSensorVSta_V>"
  UnitConverter_13/1 -> bus_creator/13  "VINP_ZFRBCMLightSensorVSta_V"
  bus_selector_1/9 -> UnitConverter_14/1  "<VINP_ZFRBCMPLampSta_flg>"
  UnitConverter_14/1 -> bus_creator/14  "VINP_ZFRBCMPLampSta_flg"
  bus_selector_1/10 -> UnitConverter_15/1  "<VINP_ZFRBCMRFTurnLpCSta_A>"
  UnitConverter_15/1 -> bus_creator/15  "VINP_ZFRBCMRFTurnLpCSta_A"
  bus_selector_1/11 -> UnitConverter_16/1  "<VINP_ZFRBCMRFogLpSWSta_flg>"
  UnitConverter_16/1 -> bus_creator/16  "VINP_ZFRBCMRFogLpSWSta_flg"
  bus_selector_1/12 -> UnitConverter_17/1  "<VINP_ZFRBCMSeatbeltSta_flg>"
  UnitConverter_17/1 -> bus_creator/17  "VINP_ZFRBCMSeatbeltSta_flg"
  bus_selector_1/13 -> UnitConverter_18/1  "<VINP_ZFRBCMWasherSWSta_flg>"
  UnitConverter_18/1 -> bus_creator/18  "VINP_ZFRBCMWasherSWSta_flg"
  bus_selector_1/14 -> UnitConverter_19/1  "<VINP_ZFRBCMWiperASSta_flg>"
  UnitConverter_19/1 -> bus_creator/19  "VINP_ZFRBCMWiperASSta_flg"
  bus_selector_1/15 -> UnitConverter_20/1  "<VINP_ZFRBCMWiperHSWSta_flg>"
  UnitConverter_20/1 -> bus_creator/20  "VINP_ZFRBCMWiperHSWSta_flg"
  bus_selector_1/16 -> UnitConverter_21/1  "<VINP_ZFRBCMWiperLSWSta_flg>"
  UnitConverter_21/1 -> bus_creator/21  "VINP_ZFRBCMWiperLSWSta_flg"
  bus_selector_1/17 -> UnitConverter_22/1  "<VINP_ZRRBCMAllDoorSta_enum>"
  UnitConverter_22/1 -> bus_creator/22  "VINP_ZRRBCMAllDoorSta_enum"
  bus_selector_1/18 -> UnitConverter_23/1  "<VINP_AirPressurePC3_kPa>"
  UnitConverter_23/1 -> bus_creator/23  "VINP_AirPressurePC3_kPa"
  bus_selector_1/19 -> UnitConverter_24/1  "<VINP_AirPressureRC1_kPa>"
  UnitConverter_24/1 -> bus_creator/24  "VINP_AirPressureRC1_kPa"
  bus_selector_1/20 -> UnitConverter_25/1  "<VINP_FDCCHASSISVCUEACPressSta_flg>"
  UnitConverter_25/1 -> bus_creator/25  "VINP_FDCCHASSISVCUEACPressSta_flg"
  bus_selector_1/21 -> UnitConverter_26/1  "<VINP_ZRRBCMCallingSWSta_flg>"
  UnitConverter_26/1 -> bus_creator/26  "VINP_ZRRBCMCallingSWSta_flg"
  bus_selector_1/22 -> UnitConverter_27/1  "<VINP_ZRRBCMLRTurnLpCSta_A>"
  UnitConverter_27/1 -> bus_creator/27  "VINP_ZRRBCMLRTurnLpCSta_A"
  bus_selector_1/23 -> UnitConverter_28/1  "<VINP_ZRRBCMPLampSta_flg>"
  UnitConverter_28/1 -> bus_creator/28  "VINP_ZRRBCMPLampSta_flg"
  bus_selector_1/24 -> UnitConverter_29/1  "<VINP_ZRRBCMRRTurnLpCSta_A>"
  UnitConverter_29/1 -> bus_creator/29  "VINP_ZRRBCMRRTurnLpCSta_A"
  bus_selector_1/25 -> UnitConverter_30/1  "<VINP_ZRRBCMSTOPSW2Sta_flg>"
  UnitConverter_30/1 -> bus_creator/30  "VINP_ZRRBCMSTOPSW2Sta_flg"
  bus_selector_1/26 -> UnitConverter_31/1  "<VINP_ZRRBCMSTOPSWSta_flg>"
  UnitConverter_31/1 -> bus_creator/31  "VINP_ZRRBCMSTOPSWSta_flg"
  bus_selector_1/27 -> UnitConverter_32/1  "<VINP_DCDCEnSta_enum>"
  UnitConverter_32/1 -> bus_creator/32  "VINP_DCDCEnSta_enum"
  bus_selector_1/28 -> UnitConverter_33/1  "<VINP_DCDCErrLvSta_enum>"
  UnitConverter_33/1 -> bus_creator/33  "VINP_DCDCErrLvSta_enum"
  bus_selector_1/29 -> UnitConverter_34/1  "<VINP_DCDCOutVolSta_V>"
  UnitConverter_34/1 -> bus_creator/34  "VINP_DCDCOutVolSta_V"
  bus_selector_1/30 -> UnitConverter_35/1  "<VINP_DCDCTempSta_C>"
  UnitConverter_35/1 -> bus_creator/35  "VINP_DCDCTempSta_C"
  bus_selector_1/31 -> UnitConverter_36/1  "<VINP_EACEnSta_enum>"
  UnitConverter_36/1 -> bus_creator/36  "VINP_EACEnSta_enum"
  bus_selector_1/32 -> UnitConverter_37/1  "<VINP_EACErrLvSta_enum>"
  UnitConverter_37/1 -> bus_creator/37  "VINP_EACErrLvSta_enum"
  bus_selector_1/33 -> UnitConverter_38/1  "<VINP_EACInvTempSta_C>"
  UnitConverter_38/1 -> bus_creator/38  "VINP_EACInvTempSta_C"
  bus_selector_1/34 -> UnitConverter_39/1  "<VINP_EHPSEnSta_enum>"
  UnitConverter_39/1 -> bus_creator/39  "VINP_EHPSEnSta_enum"
  bus_selector_1/35 -> UnitConverter_40/1  "<VINP_EHPSErrLvSta_enum>"
  UnitConverter_40/1 -> bus_creator/40  "VINP_EHPSErrLvSta_enum"
  bus_selector_1/36 -> UnitConverter_41/1  "<VINP_EHPSInvTempSta_C>"
  UnitConverter_41/1 -> bus_creator/41  "VINP_EHPSInvTempSta_C"
  bus_selector_1/37 -> UnitConverter_42/1  "<VINP_EHPSMotorSpdSta_rpm>"
  UnitConverter_42/1 -> bus_creator/42  "VINP_EHPSMotorSpdSta_rpm"
  bus_selector_1/38 -> UnitConverter_43/1  "<VINP_PDUACRlySta_enum>"
  UnitConverter_43/1 -> bus_creator/43  "VINP_PDUACRlySta_enum"
  bus_selector_1/39 -> UnitConverter_44/1  "<VINP_PDUDCDCEACEHPSHVLoopSta_enum>"
  UnitConverter_44/1 -> bus_creator/44  "VINP_PDUDCDCEACEHPSHVLoopSta_enum"
  bus_selector_1/40 -> UnitConverter_45/1  "<VINP_PDUDCDCEACEHPSPreRlySta_enum>"
  UnitConverter_45/1 -> bus_creator/45  "VINP_PDUDCDCEACEHPSPreRlySta_enum"
  bus_selector_1/41 -> UnitConverter_46/1  "<VINP_PDUDCDCEACEHPSRlySta_enum>"
  UnitConverter_46/1 -> bus_creator/46  "VINP_PDUDCDCEACEHPSRlySta_enum"
  bus_selector_1/42 -> UnitConverter_47/1  "<VINP_PDUHVILSta_enum>"
  UnitConverter_47/1 -> bus_creator/47  "VINP_PDUHVILSta_enum"
  bus_selector_1/43 -> UnitConverter_48/1  "<VINP_PDUMCUHVLoopSta_enum>"
  UnitConverter_48/1 -> bus_creator/48  "VINP_PDUMCUHVLoopSta_enum"
  bus_selector_1/44 -> UnitConverter_49/1  "<VINP_PDUMCUPosRlySta_enum>"
  UnitConverter_49/1 -> bus_creator/49  "VINP_PDUMCUPosRlySta_enum"
  bus_selector_1/45 -> UnitConverter_50/1  "<VINP_PDUMCUPreRlySta_enum>"
  UnitConverter_50/1 -> bus_creator/50  "VINP_PDUMCUPreRlySta_enum"
  bus_selector_1/46 -> UnitConverter_51/1  "<VINP_PDUSelfChkSta_enum>"
  UnitConverter_51/1 -> bus_creator/51  "VINP_PDUSelfChkSta_enum"
  [inp_CanValid_bus] -> bus_selector/1
  [inp_Hal_bus] -> bus_selector_1/1
  bus_creator/1 -> BINP_outputs/1
